simulink model "model1"  (R2021b)
settings: Solver=VariableStepAuto  StartTime=0.0  StopTime=15  RelTol=1e-3
InitFcn:
  | %thong so mo hinh ly thuyet
  | mt = 0.536;          %khoi luong cua xe day
  | mp = 0.375;          %khoi luong cua tai
  | l = 0.64;               % chieu dai day
  | g = 9.81;              %gia toc trong truong
  | M=0.536;
  | m=0.375;
  | %D=0;
  | D=0.03;
  | %thong so bo dieu khien ADRC
  | %b0 =6.14/0.04;
  | b0=154;
  | 
  | sCL = -4.3;
  | Tsettle = -5.85/sCL;
  | 
  | %Tsettle = 4.5;
  | %sCL = -5.85/Tsettle;
  | 
  | Kp = (sCL)^2;
  | Kd = -2*sCL;
  | 
  | %kESO = 350; % đặt điểm cực của bộ quan sát
  | kESO=100;
  | sESO = kESO*sCL; % điểm cực của bộ quan sát
  | 
  | l1 = -3*sESO;
  | l2 = 3*(sESO^2);
  | l3 = -(sESO)^3;
  | 
  | A = [0 1 0; 0 0 1; 0 0 0];
  | B = [0; b0; 0];
  | C = [1 0 0];
  | L = [l1; l2; l3];
  | 
  | 
  | %Bo input shaping
  | w = sqrt(g/l);
  | damping_ratio = 0.01;
  | wd = w*sqrt(1-damping_ratio^2);
  | k = exp(-damping_ratio*pi/sqrt(1-damping_ratio^2));
  | 
  | %ZV
  | A1_zv = k/(k+1);
  | A2_zv = 1/(k+1);
  | t1_zv = 0;
  | t2_zv = pi/wd;
  | 
  | %ZVD
  | A1_zvd = (k^2)/((1+k)^2);
  | A2_zvd = (2*k)/((1+k)^2);
  | A3_zvd = 1/((1+k)^2);
  | t1_zvd = 0;
  | t2_zvd = pi/wd;
  | t3_zvd = 2*pi/wd;
  | 
  | %ETM4
  | m_etm4 = 0.1;
  | I_etm4 = (1+m_etm4)*k/(k^2 + (1+m_etm4)*(k^(4/3)+k^(2/3)) + m_etm4);
  | 
  | A1_etm4 = I_etm4/(1+m_etm4);
  | A2_etm4 = I_etm4/(k^(2/3));
  | A3_etm4 = I_etm4/(k^(4/3));
  | A4_etm4 = m_etm4*I_etm4/((1+m_etm4)*(k^2));
  | t1_etm4 = 0;
  | t2_etm4 = (2*pi/3)/wd;
  | t3_etm4 = (4*pi/3)/wd;
  | t4_etm4 = 2*pi/wd;
undefined symbols (not defined in the file or in its folder): D1
settings Model: Creator=Admin  LastModifiedBy=Admin

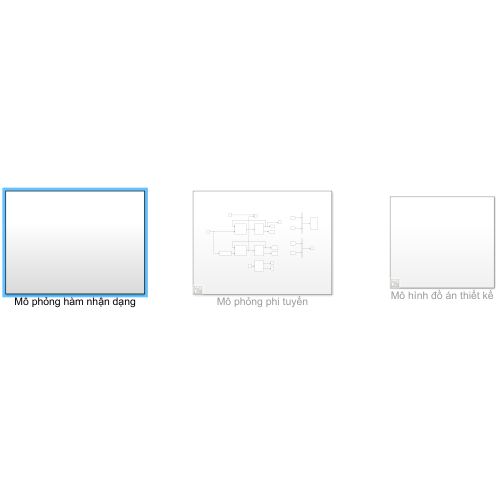
[thumbnail: Simulink's stored preview of the top-level diagram]
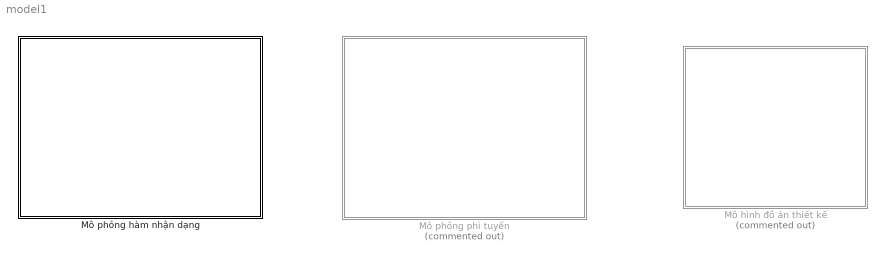
== system model1 ==
  Mô hình đồ án thiết kế : Subsystem  Commented=on
  Mô phỏng hàm nhận dạng : Subsystem
  Mô phỏng phi tuyến : Subsystem  Commented=on

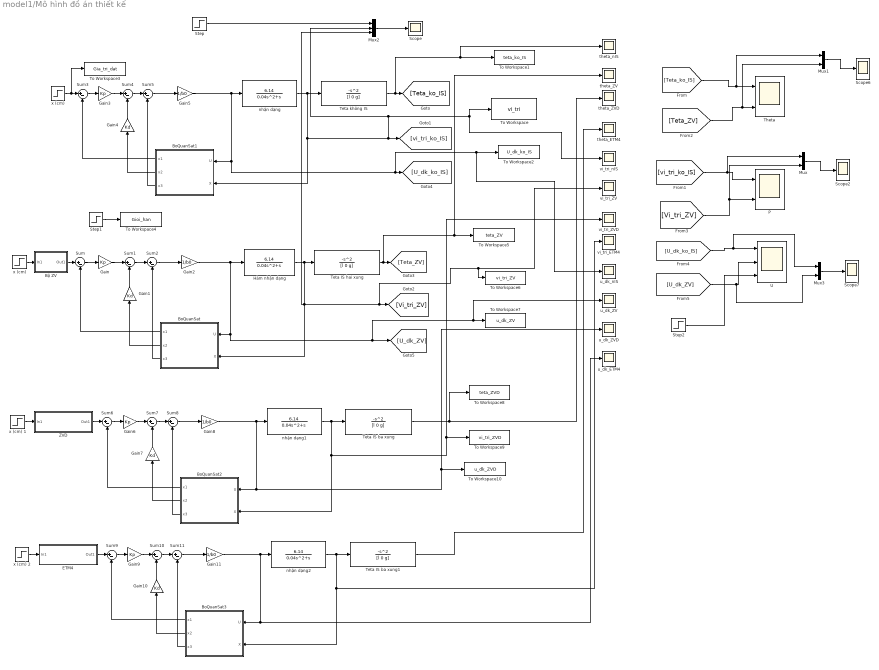
== system model1/Mô hình đồ án thiết kế ==
  " nhận dạng" : TransferFcn  Numerator=[6.14]  Denominator="[0.04 1  0]"
  " nhận dạng1" : TransferFcn  Numerator=[6.14]  Denominator="[0.04 1  0]"
  " nhận dạng2" : TransferFcn  Numerator=[6.14]  Denominator="[0.04 1  0]"
  BoQuanSat : Subsystem
  BoQuanSat1 : Subsystem
  BoQuanSat2 : Subsystem
  BoQuanSat3 : Subsystem
  Bộ ZV : Subsystem
  ETM4 : Subsystem
  Gain{,3,6,9} (4 alike) : Gain  Gain=Kp
  Gain{1,4,7,10} (4 alike) : Gain  Gain=Kd
  Gain{2,5,8,11} (4 alike) : Gain  Gain=1/b0
  Hàm nhận dạng : TransferFcn  Numerator=[6.14]  Denominator="[0.04 1  0]"
  Mux : Mux  Inputs=2
  Mux1 : Mux  Inputs=2
  Mux2 : Mux  Inputs=3
  Mux3 : Mux  Inputs=2
  P : Scope  NumInputPorts=2
  Scope{,2,6..7} (4 alike) : Scope
  Step : Step  Time=0  After=40  SampleTime=0
  Step1 : Step  Time=0  After=40  SampleTime=0
  Step2 : Step  Time=0  After=10  SampleTime=0
  Sum{,1..11} (12 alike) : Sum  Inputs=|+-
  Teta IS ba xung : TransferFcn  Numerator=[-1 0 0]  Denominator=[l 0 g]
  Teta IS ba xung1 : TransferFcn  Numerator=[-1 0 0]  Denominator=[l 0 g]
  Teta IS hai xung : TransferFcn  Numerator=[-1 0 0]  Denominator=[l 0 g]
  "Teta không IS " : TransferFcn  Numerator=[-1 0 0]  Denominator=[l 0 g]
  Theta : Scope  NumInputPorts=2
  To Workspace : ToWorkspace  VariableName=vi_tri  SaveFormat=Timeseries  SampleTime=0.005
  To Workspace1 : ToWorkspace  VariableName=teta_ko_IS  SaveFormat=Timeseries  SampleTime=-1
  To Workspace10 : ToWorkspace  VariableName=u_dk_ZVD  SaveFormat=Timeseries  SampleTime=-1
  To Workspace2 : ToWorkspace  VariableName=U_dk_ko_IS  SaveFormat=Timeseries  SampleTime=-1
  To Workspace3 : ToWorkspace  VariableName=Gia_tri_dat  SaveFormat=Timeseries  SampleTime=0.005
  To Workspace4 : ToWorkspace  VariableName=Gioi_han  SaveFormat=Timeseries  SampleTime=-1
  To Workspace5 : ToWorkspace  VariableName=teta_ZV  SaveFormat=Timeseries  SampleTime=-1
  To Workspace6 : ToWorkspace  VariableName=vi_tri_ZV  SaveFormat=Timeseries  SampleTime=-1
  To Workspace7 : ToWorkspace  VariableName=u_dk_ZV  SaveFormat=Timeseries  SampleTime=-1
  To Workspace8 : ToWorkspace  VariableName=teta_ZVD  SaveFormat=Timeseries  SampleTime=-1
  To Workspace9 : ToWorkspace  VariableName=vi_tri_ZVD  SaveFormat=Timeseries  SampleTime=-1
  U : Scope  NumInputPorts=3
  ZVD : Subsystem
  theta_ETM4 : Scope
  theta_ZV : Scope
  theta_ZVD : Scope
  theta_nIS : Scope
  u_dk_ETM4 : Scope
  u_dk_ZV : Scope
  u_dk_ZVD : Scope
  u_dk_nIS : Scope
  vi_tri_ETM4 : Scope
  vi_tri_ZV : Scope
  vi_tri_ZVD : Scope
  vi_tri_nIS : Scope
  x (cm) : Step  Time=0  After=40  SampleTime=0
  "x (cm) " : Step  Time=0  After=40  SampleTime=0
  x (cm) 1 : Step  Time=0  After=40  SampleTime=0
  x (cm) 2 : Step  Time=0  After=40  SampleTime=0
  wires:
  Gain/1 -> Sum1/1
  Sum2/1 -> Gain2/1
  BoQuanSat/2(x2) -> Gain1/1
  BoQuanSat/3(x3) -> Sum2/2
  BoQuanSat/1(x1) -> Sum/2
  Sum/1 -> Gain/1
  Sum1/1 -> Sum2/1
  Gain1/1 -> Sum1/2
  Gain2/1 -> Hàm nhận dạng/1, u_dk_ZV/1, To Workspace7/1, [U_dk_ZV], BoQuanSat/1(U)
  x (cm)/1 -> Bộ ZV/1(In1)
  Bộ ZV/1(Out1) -> Sum/1
  Gain4/1 -> Sum4/2
  Sum4/1 -> Sum5/1
  Sum5/1 -> Gain5/1
  BoQuanSat1/1(x1) -> Sum3/2
  BoQuanSat1/3(x3) -> Sum5/2
  BoQuanSat1/2(x2) -> Gain4/1
  Sum3/1 -> Gain3/1
  Gain3/1 -> Sum4/1
  Teta IS hai xung/1 -> theta_ZV/1, To Workspace5/1, [Teta_ZV]
  " nhận dạng"/1 -> "Teta không IS "/1, vi_tri_nIS/1, To Workspace/1, Mux2/2, [vi_tri_ko_IS], BoQuanSat1/2(X)
  "Teta không IS "/1 -> theta_nIS/1, To Workspace1/1, [Teta_ko_IS]
  Gain5/1 -> " nhận dạng"/1, BoQuanSat1/1(U), u_dk_nIS/1, To Workspace2/1, [U_dk_ko_IS]
  Hàm nhận dạng/1 -> Teta IS hai xung/1, vi_tri_ZV/1, To Workspace6/1, [Vi_tri_ZV], Mux2/3, BoQuanSat/2(X)
  Step/1 -> Mux2/1
  Mux2/1 -> Scope/1
  "x (cm) "/1 -> To Workspace3/1, Sum3/1
  Step1/1 -> To Workspace4/1
  [U_dk_ZV] -> Mux3/2, U/2
  Step2/1 -> U/3
  [Teta_ko_IS] -> Mux1/1, Theta/1
  [Teta_ZV] -> Mux1/2, Theta/2
  [vi_tri_ko_IS] -> Mux/1, P/1
  [Vi_tri_ZV] -> Mux/2, P/2
  Mux/1 -> Scope2/1
  Mux1/1 -> Scope6/1
  Mux3/1 -> Scope7/1
  [U_dk_ko_IS] -> Mux3/1, U/1
  BoQuanSat2/2(x2) -> Gain7/1
  Sum8/1 -> Gain8/1
  Gain8/1 -> " nhận dạng1"/1, To Workspace10/1, u_dk_ZVD/1, BoQuanSat2/1(U)
  Gain7/1 -> Sum7/2
  Sum6/1 -> Gain6/1
  BoQuanSat2/3(x3) -> Sum8/2
  Gain6/1 -> Sum7/1
  Sum7/1 -> Sum8/1
  " nhận dạng1"/1 -> Teta IS ba xung/1, BoQuanSat2/2(X), To Workspace9/1, vi_tri_ZVD/1
  BoQuanSat2/1(x1) -> Sum6/2
  ZVD/1(Out1) -> Sum6/1
  x (cm) 1/1 -> ZVD/1(In1)
  Teta IS ba xung/1 -> To Workspace8/1, theta_ZVD/1
  Teta IS ba xung1/1 -> theta_ETM4/1
  BoQuanSat3/1(x1) -> Sum9/2
  x (cm) 2/1 -> ETM4/1(In1)
  ETM4/1(Out1) -> Sum9/1
  Gain9/1 -> Sum10/1
  Sum10/1 -> Sum11/1
  Gain11/1 -> " nhận dạng2"/1, u_dk_ETM4/1, BoQuanSat3/1(U)
  BoQuanSat3/3(x3) -> Sum11/2
  Gain10/1 -> Sum10/2
  Sum9/1 -> Gain9/1
  " nhận dạng2"/1 -> Teta IS ba xung1/1, vi_tri_ETM4/1, BoQuanSat3/2(X)
  Sum11/1 -> Gain11/1
  BoQuanSat3/2(x2) -> Gain10/1

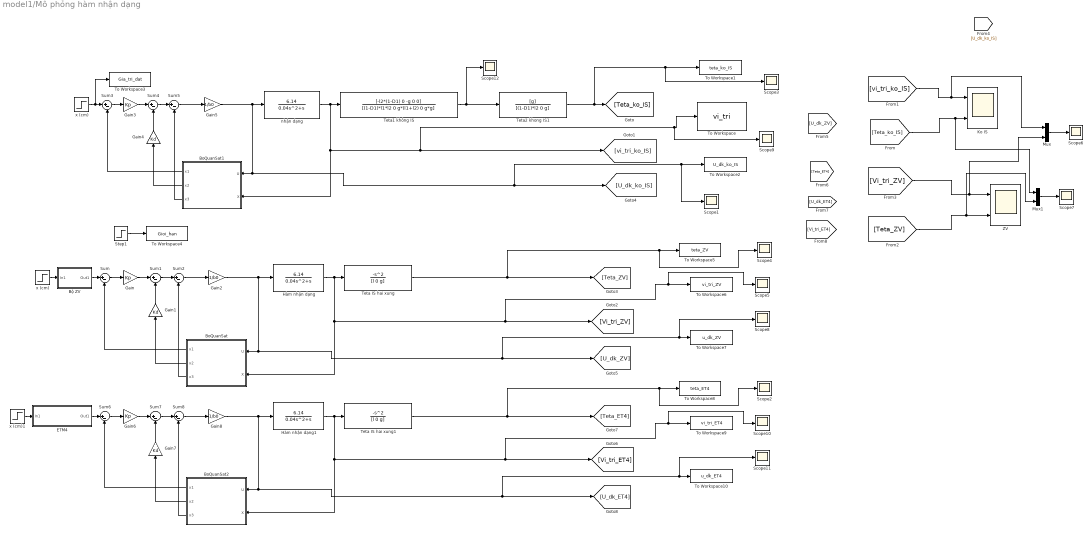
== system model1/Mô phỏng hàm nhận dạng ==
  " nhận dạng" : TransferFcn  Numerator=[6.14]  Denominator="[0.04 1  0]"
  BoQuanSat : Subsystem
  BoQuanSat1 : Subsystem
  BoQuanSat2 : Subsystem
  Bộ ZV : Subsystem
  ETM4 : Subsystem
  Gain : Gain  Gain=Kp
  Gain1 : Gain  Gain=Kd
  Gain2 : Gain  Gain=1/b0
  Gain3 : Gain  Gain=Kp
  Gain4 : Gain  Gain=Kd
  Gain5 : Gain  Gain=1/b0
  Gain6 : Gain  Gain=Kp
  Gain7 : Gain  Gain=Kd
  Gain8 : Gain  Gain=1/b0
  Hàm nhận dạng : TransferFcn  Numerator=[6.14]  Denominator="[0.04 1  0]"
  Hàm nhận dạng1 : TransferFcn  Numerator=[6.14]  Denominator="[0.04 1  0]"
  Ko IS : Scope  NumInputPorts=2
  Mux : Mux  Inputs=2
  Mux1 : Mux  Inputs=2
  Scope{1..12} (12 alike) : Scope
  Step1 : Step  Time=0  After=10  SampleTime=0
  Sum{,1..8} (9 alike) : Sum  Inputs=|+-
  Teta IS hai xung : TransferFcn  Numerator=[-1 0 0]  Denominator=[l 0 g]
  Teta IS hai xung1 : TransferFcn  Numerator=[-1 0 0]  Denominator=[l 0 g]
  "Teta1 không IS " : TransferFcn  Numerator=[-l2*(1-D1) 0 -g 0 0]  Denominator=[(1-D1)*l1*l2 0 g*(l1+l2) 0 g*g]
  Teta2 khong IS1 : TransferFcn  Numerator=[g]  Denominator=[(1-D1)*l2 0 g]
  To Workspace : ToWorkspace  VariableName=vi_tri  SaveFormat=Timeseries  SampleTime=0.005
  To Workspace1 : ToWorkspace  VariableName=teta_ko_IS  SaveFormat=Timeseries  SampleTime=-1
  To Workspace10 : ToWorkspace  VariableName=u_dk_ET4  SaveFormat=Timeseries  SampleTime=-1
  To Workspace2 : ToWorkspace  VariableName=U_dk_ko_IS  SaveFormat=Timeseries  SampleTime=-1
  To Workspace3 : ToWorkspace  VariableName=Gia_tri_dat  SaveFormat=Timeseries  SampleTime=0.005
  To Workspace4 : ToWorkspace  VariableName=Gioi_han  SaveFormat=Timeseries  SampleTime=-1
  To Workspace5 : ToWorkspace  VariableName=teta_ZV  SaveFormat=Timeseries  SampleTime=-1
  To Workspace6 : ToWorkspace  VariableName=vi_tri_ZV  SaveFormat=Timeseries  SampleTime=-1
  To Workspace7 : ToWorkspace  VariableName=u_dk_ZV  SaveFormat=Timeseries  SampleTime=-1
  To Workspace8 : ToWorkspace  VariableName=teta_ET4  SaveFormat=Timeseries  SampleTime=-1
  To Workspace9 : ToWorkspace  VariableName=vi_tri_ET4  SaveFormat=Timeseries  SampleTime=-1
  ZV : Scope  NumInputPorts=2
  x (cm) : Step  Time=0  After=50  SampleTime=0
  "x (cm) " : Step  Time=0  After=40  SampleTime=0
  x (cm)1 : Step  Time=0  After=50  SampleTime=0
  wires:
  Gain/1 -> Sum1/1
  Sum2/1 -> Gain2/1
  BoQuanSat/2(x2) -> Gain1/1
  BoQuanSat/3(x3) -> Sum2/2
  BoQuanSat/1(x1) -> Sum/2
  Sum/1 -> Gain/1
  Sum1/1 -> Sum2/1
  Gain1/1 -> Sum1/2
  Gain2/1 -> Hàm nhận dạng/1, Scope8/1, To Workspace7/1, [U_dk_ZV], BoQuanSat/1(U)
  x (cm)/1 -> Bộ ZV/1(In1)
  Bộ ZV/1(Out1) -> Sum/1
  Gain4/1 -> Sum4/2
  Sum4/1 -> Sum5/1
  Sum5/1 -> Gain5/1
  BoQuanSat1/1(x1) -> Sum3/2
  BoQuanSat1/3(x3) -> Sum5/2
  BoQuanSat1/2(x2) -> Gain4/1
  Sum3/1 -> Gain3/1
  Gain3/1 -> Sum4/1
  Teta IS hai xung/1 -> Scope4/1, To Workspace5/1, [Teta_ZV]
  [vi_tri_ko_IS] -> Mux/1, Ko IS/1
  [Vi_tri_ZV] -> Mux/2, ZV/1
  [Teta_ZV] -> Mux1/2, ZV/2
  [Teta_ko_IS] -> Mux1/1, Ko IS/2
  Mux/1 -> Scope6/1
  Mux1/1 -> Scope7/1
  " nhận dạng"/1 -> "Teta1 không IS "/1, Scope9/1, To Workspace/1, [vi_tri_ko_IS], BoQuanSat1/2(X)
  Gain5/1 -> " nhận dạng"/1, Scope1/1, To Workspace2/1, [U_dk_ko_IS], BoQuanSat1/1(U)
  Hàm nhận dạng/1 -> Teta IS hai xung/1, Scope5/1, To Workspace6/1, [Vi_tri_ZV], BoQuanSat/2(X)
  "x (cm) "/1 -> To Workspace3/1, Sum3/1
  Step1/1 -> To Workspace4/1
  BoQuanSat2/3(x3) -> Sum8/2
  Teta IS hai xung1/1 -> Scope2/1, To Workspace8/1, [Teta_ET4]
  x (cm)1/1 -> ETM4/1(In1)
  ETM4/1(Out1) -> Sum6/1
  Hàm nhận dạng1/1 -> Teta IS hai xung1/1, Scope10/1, To Workspace9/1, [Vi_tri_ET4], BoQuanSat2/2(X)
  BoQuanSat2/2(x2) -> Gain7/1
  Sum7/1 -> Sum8/1
  BoQuanSat2/1(x1) -> Sum6/2
  Sum6/1 -> Gain6/1
  Sum8/1 -> Gain8/1
  Gain6/1 -> Sum7/1
  Gain8/1 -> Hàm nhận dạng1/1, Scope11/1, To Workspace10/1, [U_dk_ET4], BoQuanSat2/1(U)
  Gain7/1 -> Sum7/2
  "Teta1 không IS "/1 -> Teta2 khong IS1/1, Scope12/1
  Teta2 khong IS1/1 -> Scope3/1, To Workspace1/1, [Teta_ko_IS]

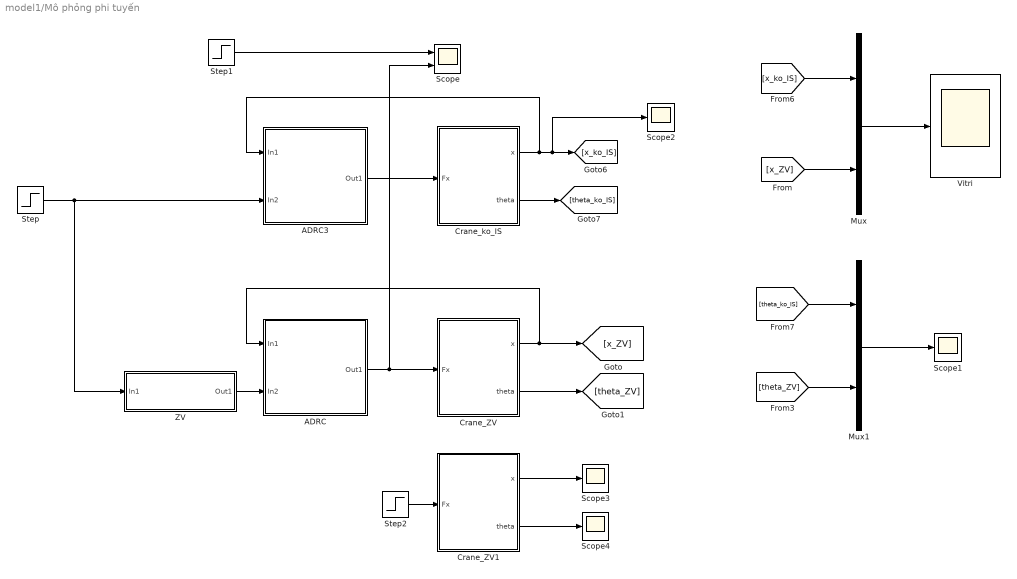
== system model1/Mô phỏng phi tuyến ==
  ADRC : Subsystem
  ADRC3 : Subsystem
  Crane_ZV : Subsystem
  Crane_ZV1 : Subsystem
  Crane_ko_IS : Subsystem
  Mux : Mux  Inputs=2
  Mux1 : Mux  Inputs=2
  Scope : Scope  NumInputPorts=2
  Scope{1..4} (4 alike) : Scope
  Step : Step  Time=0  After=40  SampleTime=0
  Step1 : Step  Time=0  After=10  SampleTime=0
  Step2 : Step  Time=0  After=40  SampleTime=0
  Vitri : Scope
  ZV : Subsystem
  wires:
  [theta_ko_IS] -> Mux1/1
  Crane_ZV/1("x ") -> ADRC/1(In1), [x_ZV]
  Crane_ZV/2(theta) -> [theta_ZV]
  Mux1/1 -> Scope1/1
  ADRC/1(Out1) -> Scope/2, Crane_ZV/1("Fx ")
  Step/1 -> ADRC3/2(In2), ZV/1(In1)
  Mux/1 -> Vitri/1
  [x_ko_IS] -> Mux/1
  Crane_ko_IS/1("x ") -> Scope2/1, [x_ko_IS], ADRC3/1(In1)
  ADRC3/1(Out1) -> Crane_ko_IS/1("Fx ")
  [theta_ZV] -> Mux1/2
  Crane_ko_IS/2(theta) -> [theta_ko_IS]
  ZV/1(Out1) -> ADRC/2(In2)
  [x_ZV] -> Mux/2
  Step1/1 -> Scope/1
  Crane_ZV1/1("x ") -> Scope3/1
  Crane_ZV1/2(theta) -> Scope4/1
  Step2/1 -> Crane_ZV1/1("Fx ")

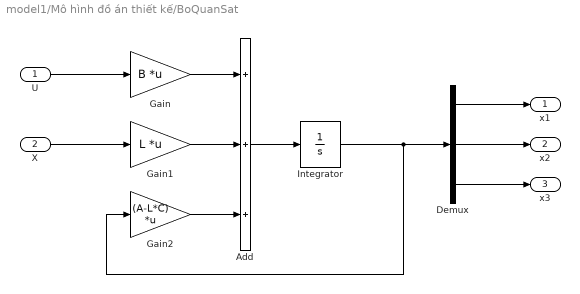
== system model1/Mô hình đồ án thiết kế/BoQuanSat ==
  U : Inport
  X : Inport  Port=2
  Add : Sum  Inputs=+++
  Demux : Demux  Outputs=3
  Gain : Gain  Gain=B  Multiplication=Matrix(K*u)
  Gain1 : Gain  Gain=L  Multiplication=Matrix(K*u)
  Gain2 : Gain  Gain=(A-L*C)  Multiplication=Matrix(K*u)
  Integrator : Integrator
  x1 : Outport
  x2 : Outport  Port=2
  x3 : Outport  Port=3
  wires:
  Demux/1 -> x1/1
  Add/1 -> Integrator/1
  Integrator/1 -> Demux/1, Gain2/1
  U/1 -> Gain/1
  Demux/3 -> x3/1
  Gain1/1 -> Add/2
  Gain2/1 -> Add/3
  X/1 -> Gain1/1
  Gain/1 -> Add/1
  Demux/2 -> x2/1

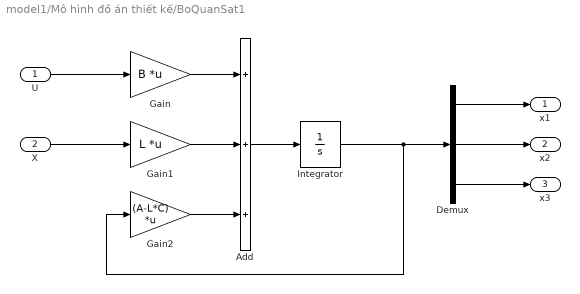
== system model1/Mô hình đồ án thiết kế/BoQuanSat1 ==
  U : Inport
  X : Inport  Port=2
  Add : Sum  Inputs=+++
  Demux : Demux  Outputs=3
  Gain : Gain  Gain=B  Multiplication=Matrix(K*u)
  Gain1 : Gain  Gain=L  Multiplication=Matrix(K*u)
  Gain2 : Gain  Gain=(A-L*C)  Multiplication=Matrix(K*u)
  Integrator : Integrator
  x1 : Outport
  x2 : Outport  Port=2
  x3 : Outport  Port=3
  wires:
  Demux/1 -> x1/1
  Add/1 -> Integrator/1
  Integrator/1 -> Demux/1, Gain2/1
  U/1 -> Gain/1
  Demux/3 -> x3/1
  Gain1/1 -> Add/2
  Gain2/1 -> Add/3
  X/1 -> Gain1/1
  Gain/1 -> Add/1
  Demux/2 -> x2/1

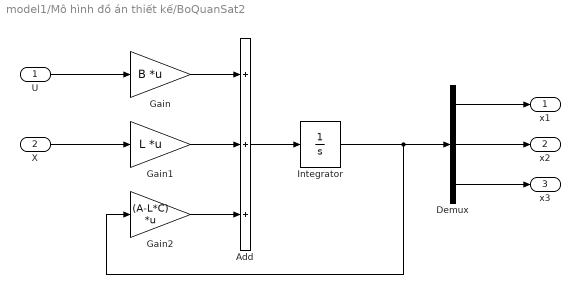
== system model1/Mô hình đồ án thiết kế/BoQuanSat2 ==
  U : Inport
  X : Inport  Port=2
  Add : Sum  Inputs=+++
  Demux : Demux  Outputs=3
  Gain : Gain  Gain=B  Multiplication=Matrix(K*u)
  Gain1 : Gain  Gain=L  Multiplication=Matrix(K*u)
  Gain2 : Gain  Gain=(A-L*C)  Multiplication=Matrix(K*u)
  Integrator : Integrator
  x1 : Outport
  x2 : Outport  Port=2
  x3 : Outport  Port=3
  wires:
  Demux/1 -> x1/1
  Add/1 -> Integrator/1
  Integrator/1 -> Demux/1, Gain2/1
  U/1 -> Gain/1
  Demux/3 -> x3/1
  Gain1/1 -> Add/2
  Gain2/1 -> Add/3
  X/1 -> Gain1/1
  Gain/1 -> Add/1
  Demux/2 -> x2/1

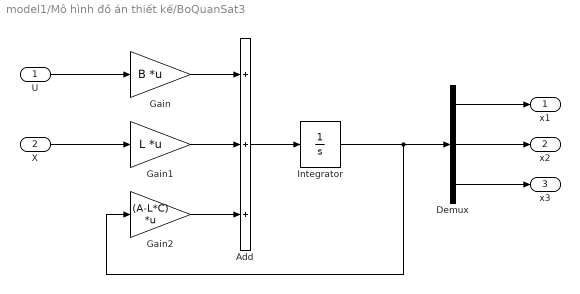
== system model1/Mô hình đồ án thiết kế/BoQuanSat3 ==
  U : Inport
  X : Inport  Port=2
  Add : Sum  Inputs=+++
  Demux : Demux  Outputs=3
  Gain : Gain  Gain=B  Multiplication=Matrix(K*u)
  Gain1 : Gain  Gain=L  Multiplication=Matrix(K*u)
  Gain2 : Gain  Gain=(A-L*C)  Multiplication=Matrix(K*u)
  Integrator : Integrator
  x1 : Outport
  x2 : Outport  Port=2
  x3 : Outport  Port=3
  wires:
  Demux/1 -> x1/1
  Add/1 -> Integrator/1
  Integrator/1 -> Demux/1, Gain2/1
  U/1 -> Gain/1
  Demux/3 -> x3/1
  Gain1/1 -> Add/2
  Gain2/1 -> Add/3
  X/1 -> Gain1/1
  Gain/1 -> Add/1
  Demux/2 -> x2/1

== system model1/Mô hình đồ án thiết kế/Bộ ZV ==
  In1 : Inport
  Gain : Gain  Gain=A1_zv
  Gain1 : Gain  Gain=A2_zv
  Sum : Sum  Inputs=|++
  Transport Delay : TransportDelay  DelayTime=t2_zv
  Out1 : Outport
  wires:
  In1/1 -> Gain1/1, Gain/1
  Gain/1 -> Sum/1
  Gain1/1 -> Transport Delay/1
  Transport Delay/1 -> Sum/2
  Sum/1 -> Out1/1

== system model1/Mô hình đồ án thiết kế/ETM4 ==
  In1 : Inport
  Gain : Gain  Gain=A1_etm4
  Gain1 : Gain  Gain=A2_etm4
  Gain2 : Gain  Gain=A3_etm4
  Gain3 : Gain  Gain=A4_etm4
  Sum : Sum  Inputs=++++
  Transport Delay : TransportDelay  DelayTime=t2_etm4
  Transport Delay1 : TransportDelay  DelayTime=t3_etm4
  Transport Delay2 : TransportDelay  DelayTime=t4_etm4
  Out1 : Outport
  wires:
  In1/1 -> Gain1/1, Gain3/1, Gain2/1, Gain/1
  Gain1/1 -> Transport Delay/1
  Transport Delay/1 -> Sum/2
  Sum/1 -> Out1/1
  Gain2/1 -> Transport Delay1/1
  Gain/1 -> Sum/1
  Transport Delay1/1 -> Sum/3
  Gain3/1 -> Transport Delay2/1
  Transport Delay2/1 -> Sum/4

== system model1/Mô hình đồ án thiết kế/ZVD ==
  In1 : Inport
  Gain : Gain  Gain=A1_zvd
  Gain1 : Gain  Gain=A2_zvd
  Gain2 : Gain  Gain=A3_zvd
  Sum : Sum  Inputs=+++
  Transport Delay : TransportDelay  DelayTime=t2_zvd
  Transport Delay1 : TransportDelay  DelayTime=t3_zvd
  Out1 : Outport
  wires:
  In1/1 -> Gain1/1, Gain2/1, Gain/1
  Gain1/1 -> Transport Delay/1
  Transport Delay/1 -> Sum/2
  Sum/1 -> Out1/1
  Gain2/1 -> Transport Delay1/1
  Gain/1 -> Sum/1
  Transport Delay1/1 -> Sum/3

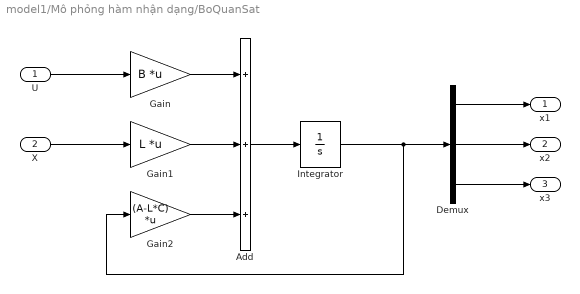
== system model1/Mô phỏng hàm nhận dạng/BoQuanSat ==
  U : Inport
  X : Inport  Port=2
  Add : Sum  Inputs=+++
  Demux : Demux  Outputs=3
  Gain : Gain  Gain=B  Multiplication=Matrix(K*u)
  Gain1 : Gain  Gain=L  Multiplication=Matrix(K*u)
  Gain2 : Gain  Gain=(A-L*C)  Multiplication=Matrix(K*u)
  Integrator : Integrator
  x1 : Outport
  x2 : Outport  Port=2
  x3 : Outport  Port=3
  wires:
  Demux/1 -> x1/1
  Add/1 -> Integrator/1
  Integrator/1 -> Demux/1, Gain2/1
  U/1 -> Gain/1
  Demux/3 -> x3/1
  Gain1/1 -> Add/2
  Gain2/1 -> Add/3
  X/1 -> Gain1/1
  Gain/1 -> Add/1
  Demux/2 -> x2/1

== system model1/Mô phỏng hàm nhận dạng/BoQuanSat1 ==
  U : Inport
  X : Inport  Port=2
  Add : Sum  Inputs=+++
  Demux : Demux  Outputs=3
  Gain : Gain  Gain=B  Multiplication=Matrix(K*u)
  Gain1 : Gain  Gain=L  Multiplication=Matrix(K*u)
  Gain2 : Gain  Gain=(A-L*C)  Multiplication=Matrix(K*u)
  Integrator : Integrator
  x1 : Outport
  x2 : Outport  Port=2
  x3 : Outport  Port=3
  wires:
  Demux/1 -> x1/1
  Add/1 -> Integrator/1
  Integrator/1 -> Demux/1, Gain2/1
  U/1 -> Gain/1
  Demux/3 -> x3/1
  Gain1/1 -> Add/2
  Gain2/1 -> Add/3
  X/1 -> Gain1/1
  Gain/1 -> Add/1
  Demux/2 -> x2/1

== system model1/Mô phỏng hàm nhận dạng/BoQuanSat2 ==
  U : Inport
  X : Inport  Port=2
  Add : Sum  Inputs=+++
  Demux : Demux  Outputs=3
  Gain : Gain  Gain=B  Multiplication=Matrix(K*u)
  Gain1 : Gain  Gain=L  Multiplication=Matrix(K*u)
  Gain2 : Gain  Gain=(A-L*C)  Multiplication=Matrix(K*u)
  Integrator : Integrator
  x1 : Outport
  x2 : Outport  Port=2
  x3 : Outport  Port=3
  wires:
  Demux/1 -> x1/1
  Add/1 -> Integrator/1
  Integrator/1 -> Demux/1, Gain2/1
  U/1 -> Gain/1
  Demux/3 -> x3/1
  Gain1/1 -> Add/2
  Gain2/1 -> Add/3
  X/1 -> Gain1/1
  Gain/1 -> Add/1
  Demux/2 -> x2/1

== system model1/Mô phỏng hàm nhận dạng/Bộ ZV ==
  In1 : Inport
  Gain : Gain  Gain=A1_zv
  Gain1 : Gain  Gain=A2_zv
  Sum : Sum  Inputs=|++
  Transport Delay : TransportDelay  DelayTime=t2_zv
  Out1 : Outport
  wires:
  In1/1 -> Gain1/1, Gain/1
  Gain/1 -> Sum/1
  Gain1/1 -> Transport Delay/1
  Transport Delay/1 -> Sum/2
  Sum/1 -> Out1/1

== system model1/Mô phỏng hàm nhận dạng/ETM4 ==
  In1 : Inport
  Gain : Gain  Gain=A1_etm4
  Gain1 : Gain  Gain=A2_etm4
  Gain2 : Gain  Gain=A3_etm4
  Gain3 : Gain  Gain=A4_etm4
  Sum : Sum  Inputs=++++
  Transport Delay : TransportDelay  DelayTime=t2_etm4
  Transport Delay1 : TransportDelay  DelayTime=t3_etm4
  Transport Delay2 : TransportDelay  DelayTime=t4_etm4
  Out1 : Outport
  wires:
  In1/1 -> Gain1/1, Gain3/1, Gain2/1, Gain/1
  Gain1/1 -> Transport Delay/1
  Transport Delay/1 -> Sum/2
  Sum/1 -> Out1/1
  Gain2/1 -> Transport Delay1/1
  Gain/1 -> Sum/1
  Transport Delay1/1 -> Sum/3
  Gain3/1 -> Transport Delay2/1
  Transport Delay2/1 -> Sum/4

== system model1/Mô phỏng phi tuyến/ADRC ==
  In1 : Inport
  In2 : Inport  Port=2
  BoQuanSat : Subsystem
  Gain : Gain  Gain=Kp
  Gain1 : Gain  Gain=Kd
  Gain2 : Gain  Gain=1/b0
  Sum : Sum  Inputs=|+-
  Sum1 : Sum  Inputs=|+-
  Sum2 : Sum  Inputs=|+-
  Out1 : Outport
  wires:
  Gain/1 -> Sum1/1
  Sum2/1 -> Gain2/1
  In2/1 -> Sum/1
  BoQuanSat/2(x2) -> Gain1/1
  BoQuanSat/3(x3) -> Sum2/2
  BoQuanSat/1(x1) -> Sum/2
  Sum/1 -> Gain/1
  Sum1/1 -> Sum2/1
  Gain1/1 -> Sum1/2
  Gain2/1 -> Out1/1, BoQuanSat/1(U(t))
  In1/1 -> BoQuanSat/2(Y(t))

== system model1/Mô phỏng phi tuyến/ADRC3 ==
  In1 : Inport
  In2 : Inport  Port=2
  BoQuanSat : Subsystem
  Gain : Gain  Gain=Kp
  Gain1 : Gain  Gain=Kd
  Gain2 : Gain  Gain=1/b0
  Sum : Sum  Inputs=|+-
  Sum1 : Sum  Inputs=|+-
  Sum2 : Sum  Inputs=|+-
  Out1 : Outport
  wires:
  Gain/1 -> Sum1/1
  Sum2/1 -> Gain2/1
  In2/1 -> Sum/1
  BoQuanSat/2(x2) -> Gain1/1
  BoQuanSat/3(x3) -> Sum2/2
  BoQuanSat/1(x1) -> Sum/2
  Sum/1 -> Gain/1
  Sum1/1 -> Sum2/1
  Gain1/1 -> Sum1/2
  Gain2/1 -> Out1/1, BoQuanSat/1(U(t))
  In1/1 -> BoQuanSat/2(Y(t))

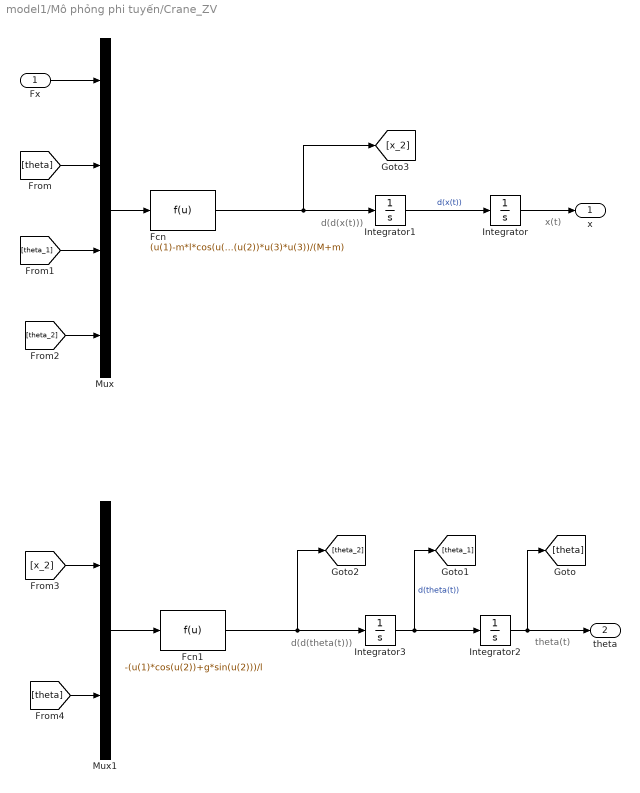
== system model1/Mô phỏng phi tuyến/Crane_ZV ==
  note: d(d(x(t)))
  note: x(t)
  note: d(d(theta(t)))
  note: theta(t)
  "Fx " : Inport
  Fcn : Fcn  Expr=(u(1)-m*l*cos(u(2))*u(4)+m*l*sin(u(2))*u(3)*u(3))/(M+m)
  Fcn1 : Fcn  Expr=-(u(1)*cos(u(2))+g*sin(u(2)))/l
  Integrator{,1..3} (4 alike) : Integrator
  Mux : Mux
  Mux1 : Mux  Inputs=2
  "x " : Outport
  theta : Outport  Port=2
  wires:
  Integrator/1 -> "x "/1
  Integrator1/1 -> Integrator/1  "d(x(t))"
  Integrator2/1 -> [theta], theta/1
  Integrator3/1 -> [theta_1], Integrator2/1  "d(theta(t))"
  Fcn/1 -> [x_2], Integrator1/1
  Mux/1 -> Fcn/1
  "Fx "/1 -> Mux/1
  [theta] -> Mux/2
  [theta_1] -> Mux/3
  [theta_2] -> Mux/4
  [x_2] -> Mux1/1
  [theta] -> Mux1/2
  Mux1/1 -> Fcn1/1
  Fcn1/1 -> [theta_2], Integrator3/1

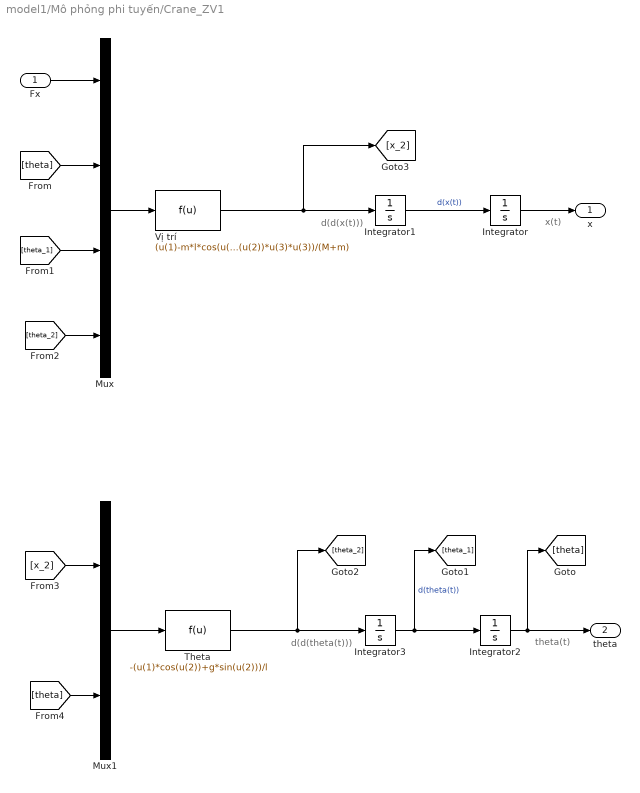
== system model1/Mô phỏng phi tuyến/Crane_ZV1 ==
  note: d(d(x(t)))
  note: x(t)
  note: d(d(theta(t)))
  note: theta(t)
  "Fx " : Inport
  Integrator{,1..3} (4 alike) : Integrator
  Mux : Mux
  Mux1 : Mux  Inputs=2
  Theta : Fcn  Expr=-(u(1)*cos(u(2))+g*sin(u(2)))/l
  Vị trí : Fcn  Expr=(u(1)-m*l*cos(u(2))*u(4)+m*l*sin(u(2))*u(3)*u(3))/(M+m)
  "x " : Outport
  theta : Outport  Port=2
  wires:
  Integrator/1 -> "x "/1
  Integrator1/1 -> Integrator/1  "d(x(t))"
  Integrator2/1 -> [theta], theta/1
  Integrator3/1 -> [theta_1], Integrator2/1  "d(theta(t))"
  Vị trí/1 -> [x_2], Integrator1/1
  Mux/1 -> Vị trí/1
  "Fx "/1 -> Mux/1
  [theta] -> Mux/2
  [theta_1] -> Mux/3
  [theta_2] -> Mux/4
  [x_2] -> Mux1/1
  [theta] -> Mux1/2
  Mux1/1 -> Theta/1
  Theta/1 -> [theta_2], Integrator3/1

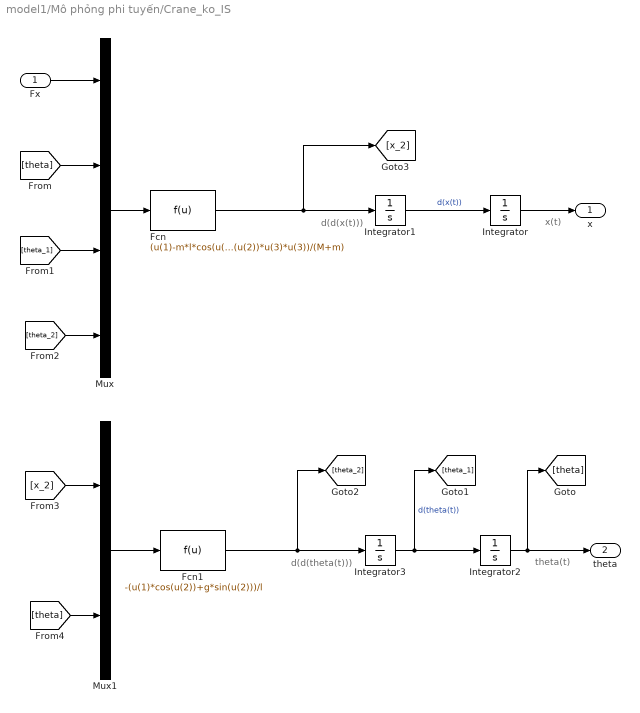
== system model1/Mô phỏng phi tuyến/Crane_ko_IS ==
  note: d(d(x(t)))
  note: x(t)
  note: d(d(theta(t)))
  note: theta(t)
  "Fx " : Inport
  Fcn : Fcn  Expr=(u(1)-m*l*cos(u(2))*u(4)+m*l*sin(u(2))*u(3)*u(3))/(M+m)
  Fcn1 : Fcn  Expr=-(u(1)*cos(u(2))+g*sin(u(2)))/l
  Integrator{,1..3} (4 alike) : Integrator
  Mux : Mux
  Mux1 : Mux  Inputs=2
  "x " : Outport
  theta : Outport  Port=2
  wires:
  Integrator/1 -> "x "/1
  Integrator1/1 -> Integrator/1  "d(x(t))"
  Integrator2/1 -> [theta], theta/1
  Integrator3/1 -> [theta_1], Integrator2/1  "d(theta(t))"
  Fcn/1 -> [x_2], Integrator1/1
  Mux/1 -> Fcn/1
  "Fx "/1 -> Mux/1
  [theta] -> Mux/2
  [theta_1] -> Mux/3
  [theta_2] -> Mux/4
  [x_2] -> Mux1/1
  [theta] -> Mux1/2
  Mux1/1 -> Fcn1/1
  Fcn1/1 -> [theta_2], Integrator3/1

== system model1/Mô phỏng phi tuyến/ZV ==
  In1 : Inport
  Gain : Gain  Gain=A1_zv
  Gain1 : Gain  Gain=A2_zv
  Sum : Sum  Inputs=|++
  Transport Delay : TransportDelay  DelayTime=t2_zv
  Out1 : Outport
  wires:
  In1/1 -> Gain1/1, Gain/1
  Gain/1 -> Sum/1
  Gain1/1 -> Transport Delay/1
  Transport Delay/1 -> Sum/2
  Sum/1 -> Out1/1

== system model1/Mô phỏng phi tuyến/ADRC/BoQuanSat ==
  U(t) : Inport
  Y(t) : Inport  Port=2
  Add : Sum  Inputs=+++
  Demux : Demux  Outputs=3
  Gain : Gain  Gain=B  Multiplication=Matrix(K*u)
  Gain1 : Gain  Gain=L  Multiplication=Matrix(K*u)
  Gain2 : Gain  Gain=(A-L*C)  Multiplication=Matrix(K*u)
  Integrator : Integrator
  x1 : Outport
  x2 : Outport  Port=2
  x3 : Outport  Port=3
  wires:
  Demux/1 -> x1/1
  Add/1 -> Integrator/1
  Integrator/1 -> Demux/1, Gain2/1
  U(t)/1 -> Gain/1
  Demux/3 -> x3/1
  Gain1/1 -> Add/2
  Gain2/1 -> Add/3
  Y(t)/1 -> Gain1/1
  Gain/1 -> Add/1
  Demux/2 -> x2/1

== system model1/Mô phỏng phi tuyến/ADRC3/BoQuanSat ==
  U(t) : Inport
  Y(t) : Inport  Port=2
  Add : Sum  Inputs=+++
  Demux : Demux  Outputs=3
  Gain : Gain  Gain=B  Multiplication=Matrix(K*u)
  Gain1 : Gain  Gain=L  Multiplication=Matrix(K*u)
  Gain2 : Gain  Gain=(A-L*C)  Multiplication=Matrix(K*u)
  Integrator : Integrator
  x1 : Outport
  x2 : Outport  Port=2
  x3 : Outport  Port=3
  wires:
  Demux/1 -> x1/1
  Add/1 -> Integrator/1
  Integrator/1 -> Demux/1, Gain2/1
  U(t)/1 -> Gain/1
  Demux/3 -> x3/1
  Gain1/1 -> Add/2
  Gain2/1 -> Add/3
  Y(t)/1 -> Gain1/1
  Gain/1 -> Add/1
  Demux/2 -> x2/1
